simulink model "lab2_pre1"  (R2023b)
settings: Solver=VariableStepAuto  StartTime=0.0  StopTime=10.0  MaxStep=2^-7  RelTol=1e-3
settings Model: Creator=insomnia  LastModifiedBy=insomnia

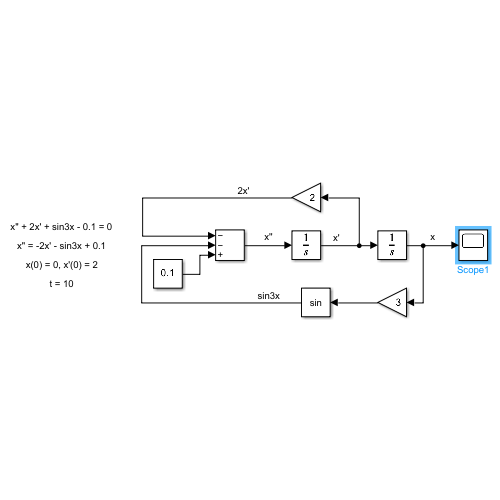
[thumbnail: Simulink's stored preview of the top-level diagram]
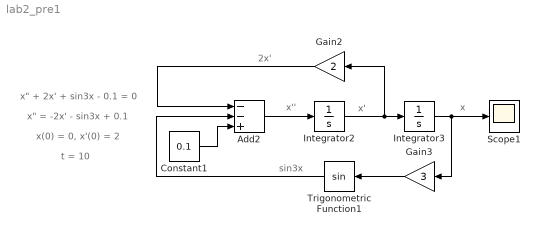
== system lab2_pre1 ==
  note: x" + 2x' + sin3x - 0.1 = 0
  note: 2x'
  note: t = 10
  note: x(0) = 0, x'(0) = 2
  note: x" = -2x' - sin3x + 0.1
  note: sin3x
  note: x'
  note: x
  note: x''
  Add2 : Sum  Inputs=--+
  Constant1 : Constant  Value=0.1
  Gain2 : Gain  Gain=2
  Gain3 : Gain  Gain=3
  Integrator2 : Integrator  InitialCondition=2
  Integrator3 : Integrator
  Scope1 : Scope
  Trigonometric Function1 : Trigonometry
  wires:
  Integrator3/1 -> Gain3/1, Scope1/1
  Gain3/1 -> Trigonometric Function1/1
  Trigonometric Function1/1 -> Add2/2
  Constant1/1 -> Add2/3
  Gain2/1 -> Add2/1
  Integrator2/1 -> Gain2/1, Integrator3/1
  Add2/1 -> Integrator2/1
